simulink model "HEMS_part"  (R2016a)
settings: Solver=ode45  StartTime=8120  StopTime=9020  RelTol=1e-3
values from neighbouring files (symbols this model uses):
  C_Batt = my_params.Cap_bat*1e3    [parameters_balanc.m]
  fo_mec = fo/pole_pairs    (= 25)    [parameters_balanc.m]
  J_Dies_u = 75    [parameters_balanc.m]
  K_freg = P_nom_u_GS*Rendiment_viscos/(2*pi*50)^2    [parameters_balanc.m]
  Ki = 500*2    (= 1000)    [parameters_balanc.m]
  Kp = 160*2    (= 320)    [parameters_balanc.m]
  P_inv_bat = my_params.P_bat_max*1e3    [parameters_balanc.m]
  P_inv_PV = my_params.P_PV_inst*1e3    [parameters_balanc.m]
  P_nom_u_GS = my_params.P_dies_max*1e3    [parameters_balanc.m]
  pole_pairs = 2    [parameters_balanc.m]
  SOC_o = my_params.SOC_init+4.2197e-04    [parameters_balanc.m]
  tao3 = 0.01    [parameters_balanc.m]
  tau_Conv_Bat = 0.01    [parameters_balanc.m]
  tau_PV = 0.01    [parameters_balanc.m]
undefined symbols (not defined in the file): C100, C20, C5
libraries: simulink x4, cstblocks x2
settings Model: PauseTimes=8  Creator=Andreu  LastModifiedBy=Milan
settings SolverCC: ZeroCrossAlgorithm=Adaptive
settings DataIOCC: FinalStateName=prev_st  InitialState=prev_st  LimitDataPoints=on  LoadInitialState=on  SaveFinalState=on  SaveFormat=Array  SignalLoggingSaveFormat=ModelDataLogs
settings DebuggingCC: MultiTaskDSMMsg=warning  MultiTaskCondExecSysMsg=none
settings HardwareCC: ProdBitPerPointer=32  ProdLargestAtomicFloat=None  ProdIntDivRoundTo=Undefined  ProdEndianess=Unspecified  ProdWordSize=32  ProdHWDeviceType=32-bit Generic
settings ModelReferenceCC: PropagateSignalLabelsOutOfModel=off
settings ConfigComp: CovModelRefEnable=Off  CovSFcnEnable=off

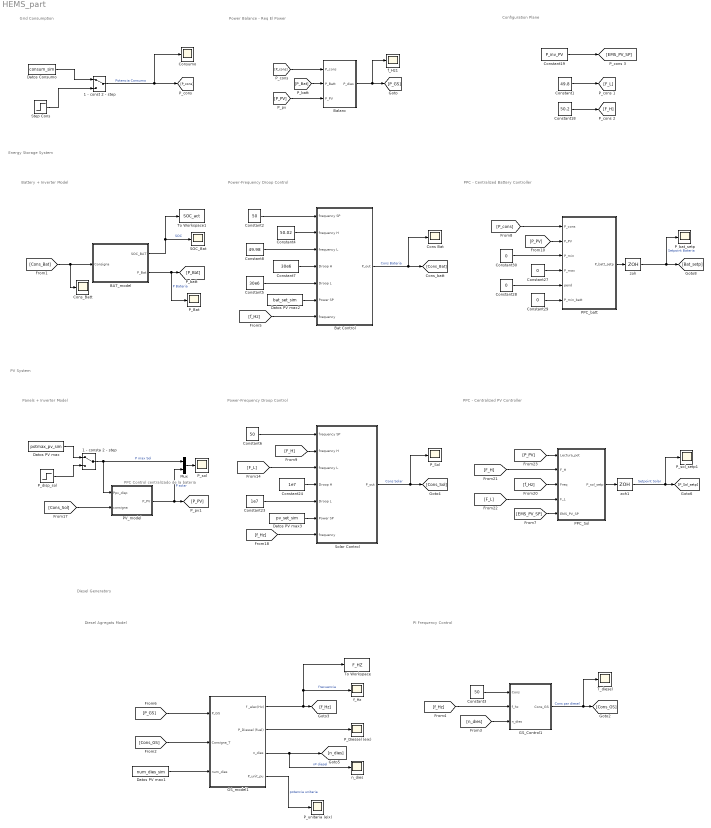
== system HEMS_part ==
  note: Grid Consumption
  note: Power Balance - Req El Power
  note: Energy Storage System
  note: PPC - Centralized Battery Controller
  note: Power-Frequency Droop Control
  note: Battery + Inverter Model
  note: PV System
  note: PPC - Centralized PV Controller
  note: Power-Frequency Droop Control
  note: Panels + Inverter Model
  note: Diesel Generators
  note: PPC Control centralizado de la bateria
  note: PI Frequency Control
  note: Diesel Agregats Model
  note: Configuration Plane
  1 - const 2 - step : ManualSwitch
  1 - consta 2 - step : ManualSwitch
  BAT_model : Subsystem
  Balanc : Subsystem
  Bat Control : Subsystem
  Cons Bat : Scope
  Cons_Batt : Scope
  Constant1 : Constant  Value=49.8
  Constant18 : Constant  Value=50.2
  Constant19 : Constant  Value=P_inv_PV
  Constant2 : Constant  Value=50
  Constant23 : Constant  Value=1e7
  Constant24 : Constant  Value=1e7
  Constant{27..30} (4 alike) : Constant  Value=0
  Constant3 : Constant  Value=50
  Constant4 : Constant  Value=50.02
  Constant5 : Constant  Value=30e6
  Constant6 : Constant  Value=50
  Constant7 : Constant  Value=30e6
  Constant8 : Constant  Value=49.98
  "Consumo " : Scope
  Datos Consumo : FromWorkspace  VariableName=consum_sim
  Datos PV max : FromWorkspace  VariableName=potmax_pv_sim
  Datos PV max1 : FromWorkspace  VariableName=num_dies_sim
  Datos PV max2 : FromWorkspace  VariableName=bat_set_sim
  Datos PV max3 : FromWorkspace  VariableName=pv_set_sim
  GS_Control1 : Subsystem
  GS_model1 : Subsystem
  Mux : Mux  Inputs=2
  PPC_Sol : Subsystem
  PPC_batt : Subsystem
  PV_model : Subsystem
  P_Bat : Scope
  P_Diessel (eix) : Scope
  P_Sol : Scope
  P_bat_setp : Scope
  P_disp_sol : Step  Time=11  Before=P_nom_u_GS*2  After=P_nom_u_GS  SampleTime=0
  P_sol : Scope
  P_sol_setp1 : Scope
  P_unitaria (eix) : Scope
  SOC_Bat : Scope
  Solar Control : Subsystem
  Step Cons : Step  Time=11  Before=P_nom_u_GS*1  After=P_nom_u_GS*1.5  SampleTime=0
  T_diesel : Scope
  To Workspace : ToWorkspace  VariableName=F_HZ  SaveFormat=Timeseries  SampleTime=-1
  To Workspace1 : ToWorkspace  VariableName=SOC_act  SaveFormat=Timeseries  SampleTime=-1
  f_Hz : Scope
  f_Hz1 : Scope
  n_dies : Scope
  zoh : ZeroOrderHold
  zoh1 : ZeroOrderHold
  wires:
  BAT_model/1(SOC_BAT) -> To Workspace1/1, SOC_Bat/1  "SOC"
  [Cons_GS] -> GS_model1/2("Consigna_T ")
  GS_model1/1(f _elec(Hz)) -> f_Hz/1, To Workspace/1, [f_Hz]  "frecuencia"
  Constant3/1 -> GS_Control1/1(Cons)
  [f_Hz] -> GS_Control1/2(f_hz)
  GS_Control1/1(Cons_GS) -> [Cons_GS], T_diesel/1  "Cons par diesel"
  [P_GS] -> GS_model1/1(P_GS)
  Bat Control/1(P_out) -> Cons Bat/1, [Cons_Bat]  "Cons Bateria"
  Constant2/1 -> Bat Control/1(frequency SP)
  Constant4/1 -> Bat Control/2(frequency H)
  Constant8/1 -> Bat Control/3(frequency L)
  Constant7/1 -> Bat Control/4(Droop H)
  Constant5/1 -> Bat Control/5(Droop L)
  Datos PV max2/1 -> Bat Control/6(Power SP)
  GS_model1/2(P_Diessel (fuel)) -> P_Diessel (eix)/1
  BAT_model/2(P_Bat) -> [P_Bat], P_Bat/1  "P Bateria"
  GS_model1/3(n_dies) -> n_dies/1, [n_dies]  "nº diesel"
  [n_dies] -> GS_Control1/3(n_dies)
  GS_model1/4(P_unit_pu) -> P_unitaria (eix)/1  "potencia unitaria"
  [P_PV] -> PPC_batt/2(P_PV)
  [P_cons] -> PPC_batt/1(P_cons)
  Constant30/1 -> PPC_batt/3(P_min)
  Constant27/1 -> PPC_batt/4(P_max)
  Constant28/1 -> PPC_batt/5(pend)
  Constant29/1 -> PPC_batt/6(P_min_batt)
  PPC_batt/1(P_batt_setp) -> zoh/1
  Balanc/1(P_dies) -> [P_GS], f_Hz1/1
  [P_Bat] -> Balanc/2(P_Batt)
  [P_PV] -> Balanc/3(P_PV)
  [P_cons] -> Balanc/1(P_cons)
  zoh/1 -> [Bat_setp], P_bat_setp/1  "Setpoint Bateria"
  Constant6/1 -> Solar Control/1(frequency SP)
  [F_H] -> Solar Control/2(frequency H)
  [F_L] -> Solar Control/3(frequency L)
  Constant24/1 -> Solar Control/4(Droop H)
  Constant23/1 -> Solar Control/5(Droop L)
  Solar Control/1(P_out) -> P_Sol/1, [Cons_Sol]  "Cons Solar"
  PV_model/1(P_PV) -> Mux/2, [P_PV]  "P solar"
  Datos PV max3/1 -> Solar Control/6(Power SP)
  [f_Hz] -> Solar Control/7(frequency)
  [P_PV] -> PPC_Sol/1(Lectura_pot)
  [F_H] -> PPC_Sol/2(F_H)
  [f_Hz] -> PPC_Sol/3(Freq)
  [F_L] -> PPC_Sol/4(F_L)
  [EMS_PV_SP] -> PPC_Sol/5(EMS_PV_SP)
  PPC_Sol/1(P_sol_setp) -> zoh1/1
  zoh1/1 -> [P_Sol_setp], P_sol_setp1/1  "Setpoint Solar"
  Mux/1 -> P_sol/1
  1 - consta 2 - step/1 -> PV_model/1("Ppv_disp "), Mux/1  "P max Sol"
  [Cons_Bat] -> BAT_model/1("Consigna "), Cons_Batt/1
  1 - const 2 - step/1 -> [P_cons], "Consumo "/1  "Potencia Consumo"
  [Cons_Sol] -> PV_model/2("consigna ")
  [f_Hz] -> Bat Control/7(frequency)
  Datos Consumo/1 -> 1 - const 2 - step/1
  Step Cons/1 -> 1 - const 2 - step/2
  Datos PV max/1 -> 1 - consta 2 - step/1
  P_disp_sol/1 -> 1 - consta 2 - step/2
  Constant1/1 -> [F_L]
  Constant18/1 -> [F_H]
  Constant19/1 -> [EMS_PV_SP]
  Datos PV max1/1 -> GS_model1/3(num_dies)

== system HEMS_part/BAT_model ==
  "Consigna " : Inport
  Bat power : Subsystem
  SOC_model : Subsystem  mask{C5=C5, C20=C20, C100=C100, SOC_o=SOC_o}
      mask prompts: C5 "C5 (Ah)"; C20 "C20 (Ah)"; C100 "C100 (Ah)"; SOC_o "SOC_o (pu)"
  SOC_BAT : Outport
  P_Bat : Outport  Port=2
  wires:
  Bat power/1(Power) -> SOC_model/1(Power), P_Bat/1
  "Consigna "/1 -> Bat power/1(Consigna)
  SOC_model/1(SOC) -> Bat power/2(SOC), SOC_BAT/1

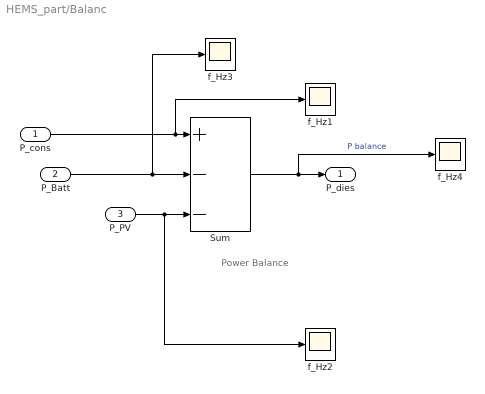
== system HEMS_part/Balanc ==
  note: Power Balance
  P_cons : Inport
  P_Batt : Inport  Port=2
  P_PV : Inport  Port=3
  Sum : Sum  Inputs=+--
  f_Hz{1..4} (4 alike) : Scope
  P_dies : Outport
  wires:
  P_cons/1 -> f_Hz1/1, Sum/1
  Sum/1 -> f_Hz4/1, P_dies/1  "P balance"
  P_Batt/1 -> Sum/2, f_Hz3/1
  P_PV/1 -> f_Hz2/1, Sum/3

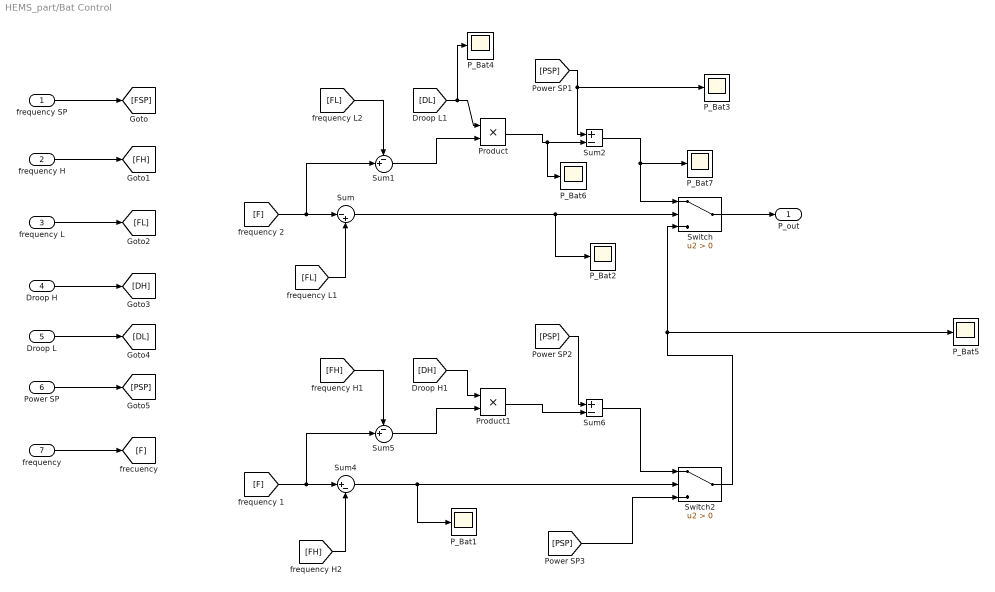
== system HEMS_part/Bat Control ==
  frequency SP : Inport
  frequency H : Inport  Port=2
  frequency L : Inport  Port=3
  Droop H : Inport  Port=4
  Droop L : Inport  Port=5
  Power SP : Inport  Port=6
  frequency : Inport  Port=7
  P_Bat{1..7} (7 alike) : Scope
  Product : Product
  Product1 : Product
  Sum : Sum  Inputs=|-+
  Sum1 : Sum  Inputs=-+|
  Sum2 : Sum  Inputs=+-
  Sum4 : Sum  Inputs=|+-
  Sum5 : Sum  Inputs=-+|
  Sum6 : Sum  Inputs=+-
  Switch : Switch  Criteria=u2 > Threshold
  Switch2 : Switch  Criteria=u2 > Threshold
  P_out : Outport
  wires:
  frequency/1 -> [F]
  Power SP/1 -> [PSP]
  Droop L/1 -> [DL]
  Droop H/1 -> [DH]
  frequency L/1 -> [FL]
  frequency H/1 -> [FH]
  frequency SP/1 -> [FSP]
  Switch/1 -> P_out/1
  [PSP] -> Sum6/1
  Switch2/1 -> P_Bat5/1, Switch/3
  [PSP] -> Switch2/3
  Sum1/1 -> Product/2
  Sum2/1 -> Switch/1, P_Bat7/1
  [FL] -> Sum1/1
  [F] -> Sum/1, Sum1/2
  [DL] -> Product/1, P_Bat4/1
  Product/1 -> Sum2/2, P_Bat6/1
  [PSP] -> Sum2/1, P_Bat3/1
  Sum/1 -> Switch/2, P_Bat2/1
  [FL] -> Sum/2
  [DH] -> Product1/1
  [FH] -> Sum5/1
  Sum4/1 -> Switch2/2, P_Bat1/1
  [FH] -> Sum4/2
  [F] -> Sum5/2, Sum4/1
  Sum6/1 -> Switch2/1
  Product1/1 -> Sum6/2
  Sum5/1 -> Product1/2

== system HEMS_part/GS_Control1 ==
  Cons : Inport
  f_hz : Inport  Port=2
  n_dies : Inport  Port=3
  Filter : TransferFcn  Denominator=[tao3 1]
  Gain : Gain  Gain=2*pi
  Gain1 : Gain  Gain=P_nom_u_GS/2/pi/50
  PID_aw : Subsystem
  Sum1 : Sum  Inputs=|+-
  Cons_GS : Outport
  wires:
  Gain1/1 -> PID_aw/2(saturacio)
  n_dies/1 -> Gain1/1
  Filter/1 -> PID_aw/1(senyal)
  PID_aw/1(sortida) -> Cons_GS/1
  Gain/1 -> Filter/1
  f_hz/1 -> Sum1/2
  Cons/1 -> Sum1/1
  Sum1/1 -> Gain/1

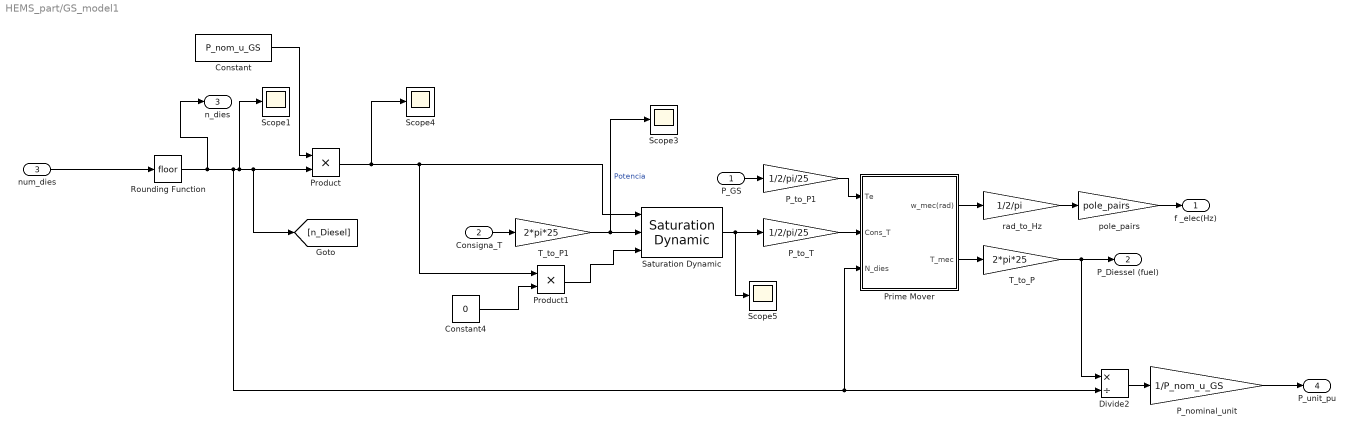
== system HEMS_part/GS_model1 ==
  P_GS : Inport
  "Consigna_T " : Inport  Port=2
  num_dies : Inport  Port=3
  Constant : Constant  Value=P_nom_u_GS
  Constant4 : Constant  Value=0
  Divide2 : Product  Inputs=*/
  P_nominal_unit : Gain  Gain=1/P_nom_u_GS
  P_to_P1 : Gain  Gain=1/2/pi/25
  P_to_T : Gain  Gain=1/2/pi/25
  Prime Mover : Subsystem
  Product : Product
  Product1 : Product
  Rounding Function : Rounding
  Saturation Dynamic : simulink/Discontinuities/Saturation Dynamic  OutMin=[]  OutMax=[]  OutDataTypeStr=Inherit: Same as second input  OutDataType=fixdt(1, 16)  OutScaling=2^-10  DoSatur=off
  Scope{1,3..5} (4 alike) : Scope
  T_to_P : Gain  Gain=2*pi*25
  T_to_P1 : Gain  Gain=2*pi*25
  pole_pairs : Gain  Gain=pole_pairs
  rad_to_Hz : Gain  Gain=1/2/pi
  f _elec(Hz) : Outport
  P_Diessel (fuel) : Outport  Port=2
  n_dies : Outport  Port=3
  P_unit_pu : Outport  Port=4
  wires:
  P_GS/1 -> P_to_P1/1
  Saturation Dynamic/1 -> Scope5/1, P_to_T/1
  Prime Mover/1(w_mec(rad)) -> rad_to_Hz/1
  Constant/1 -> Product/1
  Rounding Function/1 -> n_dies/1, Divide2/2, Prime Mover/3(N_dies), Scope1/1, [n_Diesel], Product/2
  Constant4/1 -> Product1/2
  Product1/1 -> Saturation Dynamic/3
  num_dies/1 -> Rounding Function/1
  "Consigna_T "/1 -> T_to_P1/1
  T_to_P1/1 -> Scope3/1, Saturation Dynamic/2  "Potencia"
  P_to_T/1 -> Prime Mover/2(Cons_T)
  P_to_P1/1 -> Prime Mover/1(Te)
  Prime Mover/2(T_mec) -> T_to_P/1
  T_to_P/1 -> Divide2/1, P_Diessel (fuel)/1
  rad_to_Hz/1 -> pole_pairs/1
  Divide2/1 -> P_nominal_unit/1
  P_nominal_unit/1 -> P_unit_pu/1
  pole_pairs/1 -> f _elec(Hz)/1
  Product/1 -> Scope4/1, Product1/1, Saturation Dynamic/1

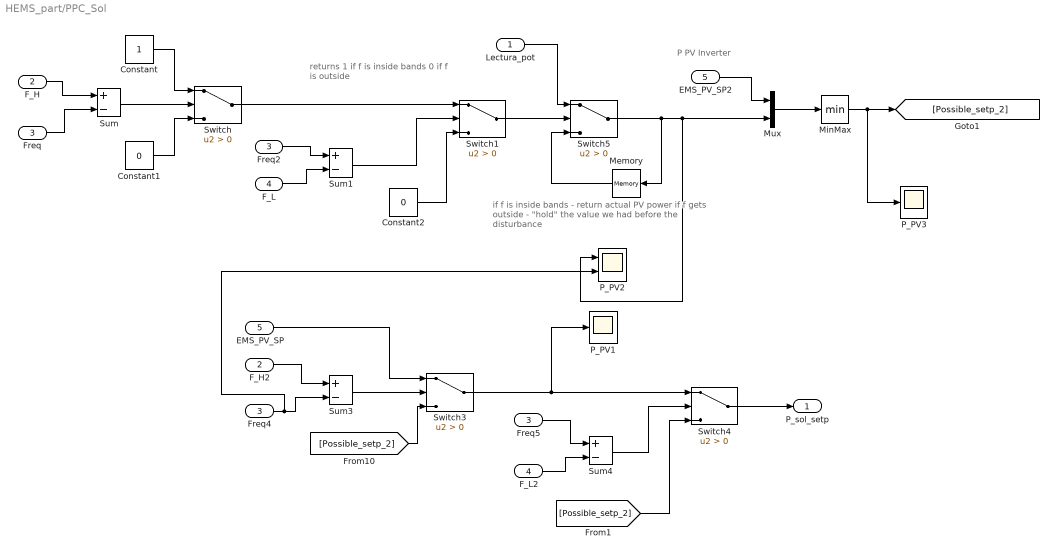
== system HEMS_part/PPC_Sol ==
  note: P PV Inverter
  note: if f is inside bands -  return actual PV power
      | if f gets outside     - "hold" the value we had
      |                                before the disturbance
  note: returns 1 if f is  inside bands
      |            0 if f is outside
  Lectura_pot : Inport
  F_H : Inport  Port=2
  Freq : Inport  Port=3
  F_L : Inport  Port=4
  EMS_PV_SP : Inport  Port=5
  Constant : Constant
  Constant1 : Constant  Value=0
  Constant2 : Constant  Value=0
  EMS_PV_SP2 : InportShadow  Port=5
  F_H2 : InportShadow  Port=2
  F_L2 : InportShadow  Port=4
  Freq2 : InportShadow  Port=3
  Freq4 : InportShadow  Port=3
  Freq5 : InportShadow  Port=3
  Memory : Memory
  MinMax : MinMax
  Mux : Mux  Inputs=2
  P_PV1 : Scope
  P_PV2 : Scope  NumInputPorts=2
  P_PV3 : Scope
  Sum{,1,3..4} (4 alike) : Sum  Inputs=+-
  Switch{,1,3..5} (5 alike) : Switch  Criteria=u2 > Threshold
  P_sol_setp : Outport
  wires:
  MinMax/1 -> [Possible_setp_2], P_PV3/1
  Constant2/1 -> Switch1/3
  Constant1/1 -> Switch/3
  Constant/1 -> Switch/1
  Mux/1 -> MinMax/1
  Switch5/1 -> Memory/1, Mux/2, P_PV2/1
  EMS_PV_SP2/1 -> Mux/1
  Lectura_pot/1 -> Switch5/1
  F_H2/1 -> Sum3/1
  Switch4/1 -> P_sol_setp/1
  [Possible_setp_2] -> Switch4/3
  [Possible_setp_2] -> Switch3/3
  F_L2/1 -> Sum4/2
  Freq5/1 -> Sum4/1
  Switch3/1 -> Switch4/1, P_PV1/1
  Sum4/1 -> Switch4/2
  EMS_PV_SP/1 -> Switch3/1
  Freq4/1 -> Sum3/2, P_PV2/2
  Sum3/1 -> Switch3/2
  F_L/1 -> Sum1/2
  Freq2/1 -> Sum1/1
  Switch/1 -> Switch1/1
  Sum1/1 -> Switch1/2
  Switch1/1 -> Switch5/2
  Freq/1 -> Sum/2
  F_H/1 -> Sum/1
  Sum/1 -> Switch/2
  Memory/1 -> Switch5/3

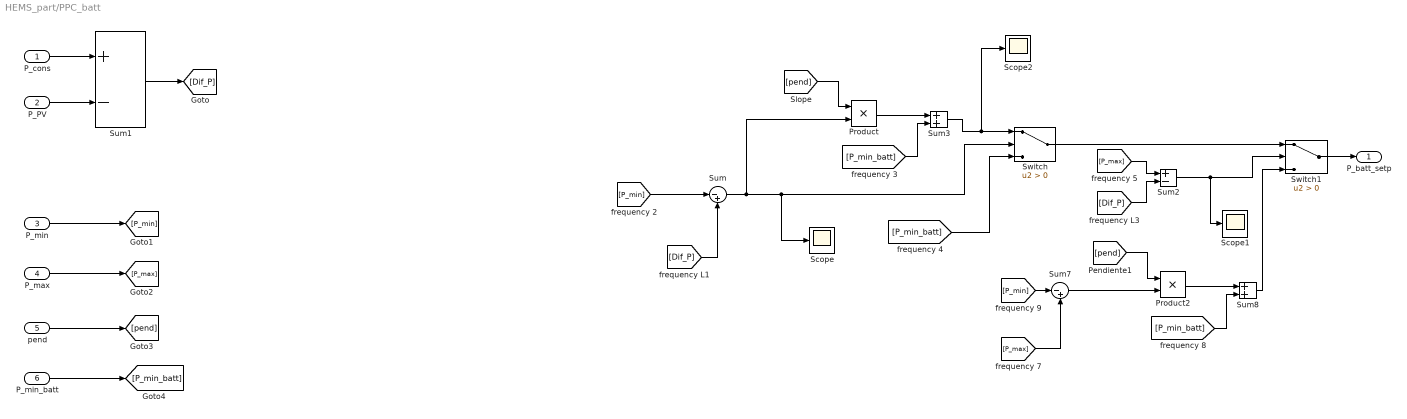
== system HEMS_part/PPC_batt ==
  P_cons : Inport
  P_PV : Inport  Port=2
  P_min : Inport  Port=3
  P_max : Inport  Port=4
  pend : Inport  Port=5
  P_min_batt : Inport  Port=6
  Product : Product
  Product2 : Product
  Scope : Scope
  Scope1 : Scope
  Scope2 : Scope
  Sum : Sum  Inputs=|-+
  Sum1 : Sum  Inputs=+-
  Sum2 : Sum  Inputs=+-
  Sum3 : Sum
  Sum7 : Sum  Inputs=|-+
  Sum8 : Sum
  Switch : Switch  Criteria=u2 > Threshold
  Switch1 : Switch  Criteria=u2 > Threshold
  P_batt_setp : Outport
  wires:
  P_PV/1 -> Sum1/2
  P_cons/1 -> Sum1/1
  Sum1/1 -> [Dif_P]
  [Dif_P] -> Sum/2
  Sum/1 -> Product/2, Scope/1, Switch/2
  [pend] -> Product/1
  Sum3/1 -> Scope2/1, Switch/1
  [P_min] -> Sum/1
  Switch/1 -> Switch1/1
  P_min/1 -> [P_min]
  P_max/1 -> [P_max]
  pend/1 -> [pend]
  P_min_batt/1 -> [P_min_batt]
  Product/1 -> Sum3/1
  [P_min_batt] -> Sum3/2
  [P_min_batt] -> Switch/3
  [Dif_P] -> Sum2/2
  [P_max] -> Sum2/1
  Sum2/1 -> Scope1/1, Switch1/2
  [pend] -> Product2/1
  Sum8/1 -> Switch1/3
  Sum7/1 -> Product2/2
  Product2/1 -> Sum8/1
  [P_min_batt] -> Sum8/2
  [P_max] -> Sum7/2
  [P_min] -> Sum7/1
  Switch1/1 -> P_batt_setp/1

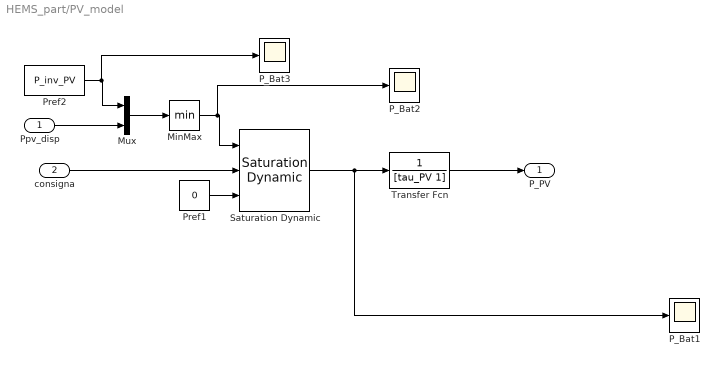
== system HEMS_part/PV_model ==
  "Ppv_disp " : Inport
  "consigna " : Inport  Port=2
  MinMax : MinMax
  Mux : Mux  Inputs=2
  P_Bat1 : Scope
  P_Bat2 : Scope
  P_Bat3 : Scope
  Pref1 : Constant  Value=0
  Pref2 : Constant  Value=P_inv_PV
  Saturation Dynamic : simulink/Discontinuities/Saturation Dynamic  OutMin=[]  OutMax=[]  OutDataTypeStr=Inherit: Same as second input  OutDataType=fixdt(1, 16)  OutScaling=2^-10  DoSatur=off
  Transfer Fcn : TransferFcn  Denominator=[tau_PV 1]
  P_PV : Outport
  wires:
  Pref1/1 -> Saturation Dynamic/3
  "consigna "/1 -> Saturation Dynamic/2
  Saturation Dynamic/1 -> P_Bat1/1, Transfer Fcn/1
  Transfer Fcn/1 -> P_PV/1
  Pref2/1 -> P_Bat3/1, Mux/1
  MinMax/1 -> P_Bat2/1, Saturation Dynamic/1
  Mux/1 -> MinMax/1
  "Ppv_disp "/1 -> Mux/2

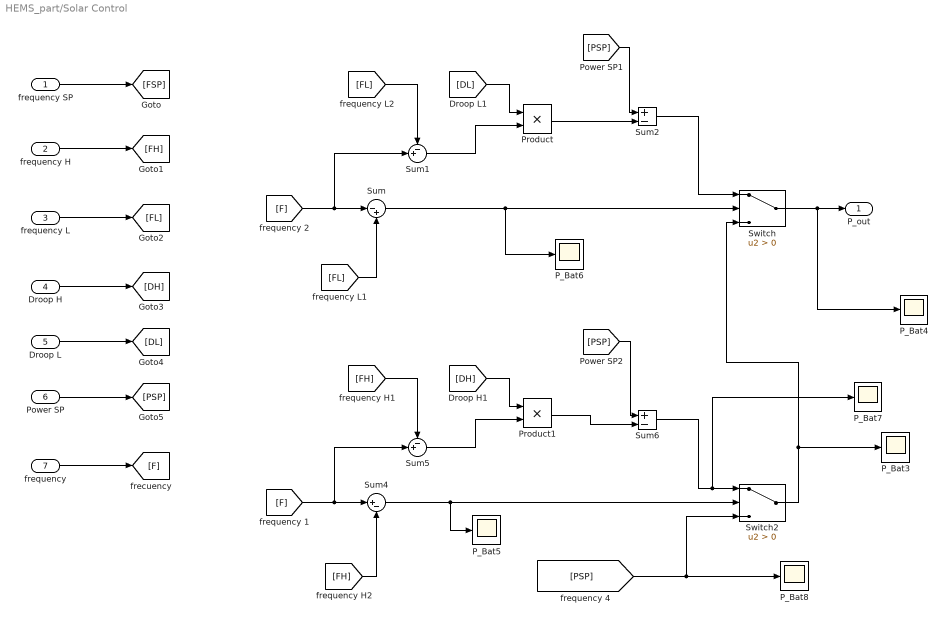
== system HEMS_part/Solar Control ==
  frequency SP : Inport
  frequency H : Inport  Port=2
  frequency L : Inport  Port=3
  Droop H : Inport  Port=4
  Droop L : Inport  Port=5
  Power SP : Inport  Port=6
  frequency : Inport  Port=7
  P_Bat{3..8} (6 alike) : Scope
  Product : Product
  Product1 : Product
  Sum : Sum  Inputs=|-+
  Sum1 : Sum  Inputs=-+|
  Sum2 : Sum  Inputs=+-
  Sum4 : Sum  Inputs=|+-
  Sum5 : Sum  Inputs=-+|
  Sum6 : Sum  Inputs=+-
  Switch : Switch  Criteria=u2 > Threshold
  Switch2 : Switch  Criteria=u2 > Threshold
  P_out : Outport
  wires:
  [PSP] -> Sum2/1
  Product/1 -> Sum2/2
  Sum2/1 -> Switch/1
  Sum/1 -> P_Bat6/1, Switch/2
  Sum5/1 -> Product1/2
  Product1/1 -> Sum6/2
  Sum6/1 -> Switch2/1, P_Bat7/1
  [F] -> Sum4/1, Sum5/2
  [FH] -> Sum4/2
  Sum4/1 -> Switch2/2, P_Bat5/1
  [FH] -> Sum5/1
  [DH] -> Product1/1
  [FL] -> Sum/2
  [DL] -> Product/1
  [F] -> Sum1/2, Sum/1
  [FL] -> Sum1/1
  Sum1/1 -> Product/2
  [PSP] -> Switch2/3, P_Bat8/1
  Switch2/1 -> Switch/3, P_Bat3/1
  [PSP] -> Sum6/1
  Switch/1 -> P_out/1, P_Bat4/1
  frequency SP/1 -> [FSP]
  frequency H/1 -> [FH]
  frequency L/1 -> [FL]
  Droop H/1 -> [DH]
  Droop L/1 -> [DL]
  Power SP/1 -> [PSP]
  frequency/1 -> [F]

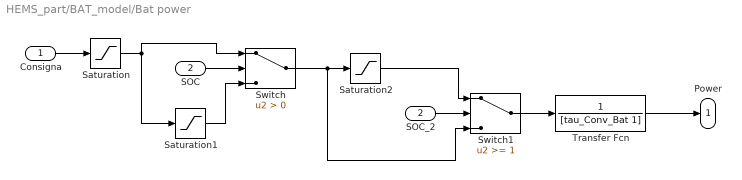
== system HEMS_part/BAT_model/Bat power ==
  Consigna : Inport
  SOC : Inport  Port=2
  SOC_2 : InportShadow  Port=2
  Saturation : Saturate  UpperLimit=P_inv_bat  LowerLimit=-P_inv_bat
  Saturation1 : Saturate  UpperLimit=0  LowerLimit=-inf
  Saturation2 : Saturate  UpperLimit=inf  LowerLimit=0
  Switch : Switch  Criteria=u2 > Threshold
  Switch1 : Switch  Threshold=1
  Transfer Fcn : TransferFcn  Denominator=[tau_Conv_Bat 1]
  Power : Outport
  wires:
  Transfer Fcn/1 -> Power/1
  Consigna/1 -> Saturation/1
  Saturation/1 -> Switch/1, Saturation1/1
  Switch/1 -> Saturation2/1, Switch1/3
  Saturation1/1 -> Switch/3
  SOC/1 -> Switch/2
  SOC_2/1 -> Switch1/2
  Saturation2/1 -> Switch1/1
  Switch1/1 -> Transfer Fcn/1

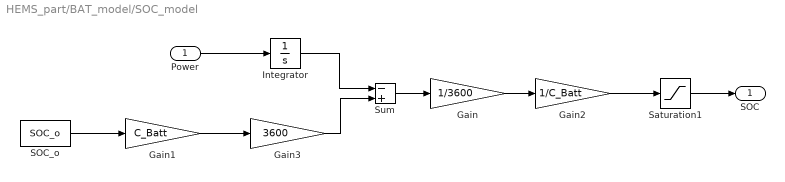
== system HEMS_part/BAT_model/SOC_model ==
  Power : Inport
  Gain : Gain  Gain=1/3600
  Gain1 : Gain  Gain=C_Batt
  Gain2 : Gain  Gain=1/C_Batt
  Gain3 : Gain  Gain=3600
  Integrator : Integrator
  SOC_o : Constant  Value=SOC_o
  Saturation1 : Saturate  UpperLimit=1  LowerLimit=0
  Sum : Sum  Inputs=-+
  SOC : Outport
  wires:
  Integrator/1 -> Sum/1
  SOC_o/1 -> Gain1/1
  Sum/1 -> Gain/1
  Power/1 -> Integrator/1
  Gain/1 -> Gain2/1
  Gain1/1 -> Gain3/1
  Gain2/1 -> Saturation1/1
  Gain3/1 -> Sum/2
  Saturation1/1 -> SOC/1

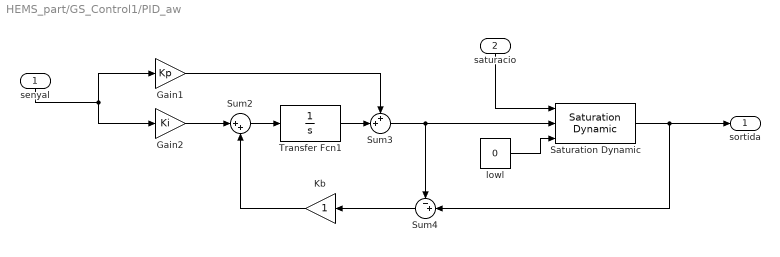
== system HEMS_part/GS_Control1/PID_aw ==
  senyal : Inport
  saturacio : Inport  Port=2
  Gain1 : Gain  Gain=Kp
  Gain2 : Gain  Gain=Ki
  Kb : Gain
  Saturation Dynamic : simulink/Discontinuities/Saturation Dynamic  OutMin=[]  OutMax=[]  OutDataTypeStr=Inherit: Same as second input  OutDataType=fixdt(1, 16)  OutScaling=2^-10  DoSatur=off
  Sum2 : Sum  Inputs=|++
  Sum3 : Sum  Inputs=++|
  Sum4 : Sum  Inputs=-+|
  Transfer Fcn1 : TransferFcn  Denominator=[1 0]
  lowl : Constant  Value=0
  sortida : Outport
  wires:
  senyal/1 -> Gain2/1, Gain1/1
  lowl/1 -> Saturation Dynamic/3
  Transfer Fcn1/1 -> Sum3/2
  Sum3/1 -> Sum4/1, Saturation Dynamic/2
  Gain1/1 -> Sum3/1
  Saturation Dynamic/1 -> Sum4/2, sortida/1
  saturacio/1 -> Saturation Dynamic/1
  Sum4/1 -> Kb/1
  Gain2/1 -> Sum2/1
  Sum2/1 -> Transfer Fcn1/1
  Kb/1 -> Sum2/2

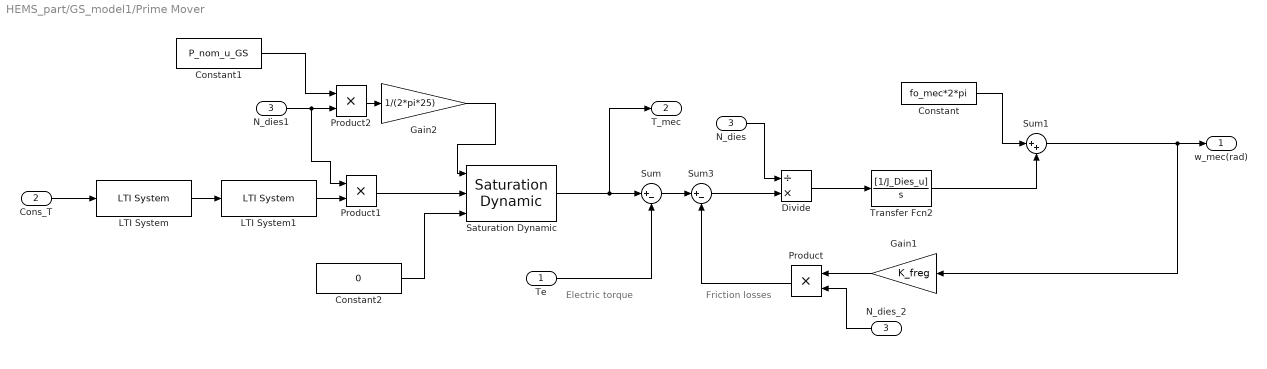
== system HEMS_part/GS_model1/Prime Mover ==
  note: Friction losses
  note: Electric torque
  Te : Inport
  Cons_T : Inport  Port=2
  N_dies : Inport  Port=3
  Constant : Constant  Value=fo_mec*2*pi
  Constant1 : Constant  Value=P_nom_u_GS
  Constant2 : Constant  Value=0
  Divide : Product  Inputs=/*
  Gain1 : Gain  Gain=K_freg
  Gain2 : Gain  Gain=1/(2*pi*25)
  LTI System : cstblocks/LTI System  sys=Actuator  IC=[]
  LTI System1 : cstblocks/LTI System  sys=Combustion  IC=[]
  N_dies1 : InportShadow  Port=3
  N_dies_2 : InportShadow  Port=3
  Product : Product
  Product1 : Product
  Product2 : Product
  Saturation Dynamic : simulink/Discontinuities/Saturation Dynamic  OutMin=[]  OutMax=[]  OutDataTypeStr=Inherit: Same as second input  OutDataType=fixdt(1, 16)  OutScaling=2^-10  DoSatur=off
  Sum : Sum  Inputs=|+-
  Sum1 : Sum  Inputs=|++
  Sum3 : Sum  Inputs=|+-
  Transfer Fcn2 : TransferFcn  Numerator=[1/J_Dies_u]  Denominator=[1 0]
  w_mec(rad) : Outport
  T_mec : Outport  Port=2
  wires:
  Te/1 -> Sum/2
  LTI System/1 -> LTI System1/1
  Cons_T/1 -> LTI System/1
  Constant/1 -> Sum1/1
  Sum/1 -> Sum3/1
  Gain1/1 -> Product/1
  Product/1 -> Sum3/2
  Sum3/1 -> Divide/2
  Divide/1 -> Transfer Fcn2/1
  N_dies/1 -> Divide/1
  N_dies_2/1 -> Product/2
  Sum1/1 -> Gain1/1, w_mec(rad)/1
  Transfer Fcn2/1 -> Sum1/2
  N_dies1/1 -> Product1/1, Product2/2
  LTI System1/1 -> Product1/2
  Product1/1 -> Saturation Dynamic/2
  Saturation Dynamic/1 -> T_mec/1, Sum/1
  Constant1/1 -> Product2/1
  Product2/1 -> Gain2/1
  Gain2/1 -> Saturation Dynamic/1
  Constant2/1 -> Saturation Dynamic/3
